simulink model "ImageProcessing"  (R2018b)
settings: Solver=FixedStepAuto  StartTime=0.0  StopTime=70  FixedStep=0.025  RelTol=1e-3  EnableMultiTasking=on
settings Model: Creator=barthal  LastModifiedBy=barthal
settings SolverCC: PositivePriorityOrder=on
settings DataIOCC: Decimation=5  SaveFormat=StructureWithTime
settings OptimizationCC: EnhancedBackFolding=on  PassReuseOutputArgsAs=Individual arguments  MaxStackSize=64  OptimizeBlockOrder=speed  DifferentSizesBufferReuse=on  OptimizationCustomize=off
settings DebuggingCC: ParameterTunabilityLossMsg=error
settings HardwareCC: ProdBitPerPointer=32  ProdBitPerSizeT=32  ProdBitPerPtrDiffT=32  ProdLargestAtomicInteger=Long  ProdLargestAtomicFloat=Double  ProdWordSize=32  ProdHWDeviceType=ARM Compatible->ARM Cortex
settings ModelReferenceCC: ModelReferenceNumInstancesAllowed=Single
settings RTWCC: SystemTargetFile=ert.tlc  HardwareBoard=Raspberry Pi  TLCOptions="-aInlineSetEventsForThisBaseRateFcn=TLC_FALSE -aSuppressMultiTaskScheduler=TLC_FALSE  -aRateBasedStepFcn=0"  GenCodeOnly=on  TemplateMakefile=ert_default_tmf  GenerateReport=on  Toolchain=GNU GCC Raspberry Pi  BuildConfiguration=Faster Runs  IncludeHyperlinkInReport=on  LaunchReport=on  TargetLang=C++  GenerateTraceInfo=on  GenerateTraceReport=on  GenerateTraceReportSl=on  GenerateTraceReportSf=on  GenerateTraceReportEml=on
settings CodeAppCC: ForceParamTrailComments=on  IgnoreCustomStorageClasses=off  OperatorAnnotations=on  SimulinkDataObjDesc=on  SFDataObjDesc=on  InsertBlockDesc=on
settings ERTTargetCC: TargetLangStandard=C++03 (ISO)  MatFileLogging=on  MultiInstanceERTCode=on  CodeInterfacePackaging=C++ class  SupportVariableSizeSignals=on  MultiInstanceErrorCode=Warning  RootIOFormat=Structure reference

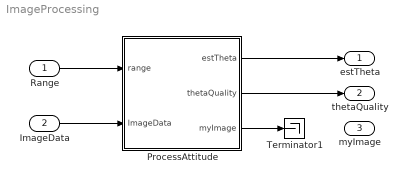
== system ImageProcessing ==
  Range : Inport  OutDataTypeStr=double  PortDimensions=4
  ImageData : Inport  Port=2  OutDataTypeStr=uint8  PortDimensions=[307200]
  ProcessAttitude : Subsystem
  Terminator1 : Terminator
  estTheta : Outport  OutDataTypeStr=double  PortDimensions=1
  thetaQuality : Outport  Port=2  OutDataTypeStr=double  PortDimensions=1
  myImage : Outport  Port=3  OutDataTypeStr=uint8
  wires:
  Range/1 -> ProcessAttitude/1(range)
  ImageData/1 -> ProcessAttitude/2(ImageData)
  ProcessAttitude/3(myImage) -> Terminator1/1
  ProcessAttitude/2(thetaQuality) -> thetaQuality/1
  ProcessAttitude/1(estTheta) -> estTheta/1

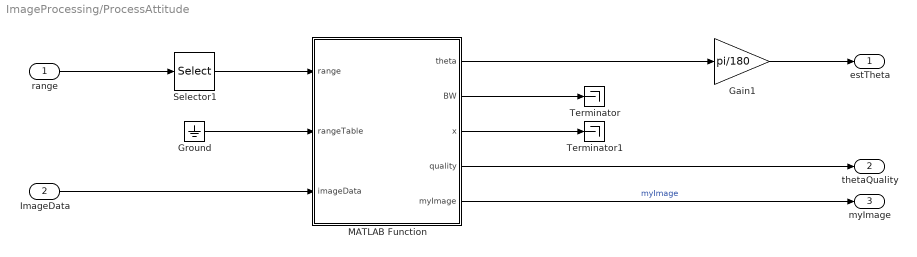
== system ImageProcessing/ProcessAttitude ==
  range : Inport  PortDimensions=4
  ImageData : Inport  Port=2  OutDataTypeStr=uint8  PortDimensions=[307200]
  Gain1 : Gain  Gain=pi/180
  Ground : Ground
  MATLAB Function : MATLAB Function  TreatAsAtomicUnit=on
  Selector1 : Selector  InputPortWidth=4  IndexOptions=Index vector (dialog)  Indices=1  OutputSizes=1
  Terminator : Terminator
  Terminator1 : Terminator
  estTheta : Outport
  thetaQuality : Outport  Port=2
  myImage : Outport  Port=3  OutDataTypeStr=uint8
  wires:
  MATLAB Function/3(x) -> Terminator1/1
  MATLAB Function/2(BW) -> Terminator/1
  MATLAB Function/5(myImage) -> myImage/1  "myImage"
  MATLAB Function/4(quality) -> thetaQuality/1
  MATLAB Function/1(theta) -> Gain1/1
  range/1 -> Selector1/1
  Selector1/1 -> MATLAB Function/1(range)
  Gain1/1 -> estTheta/1
  ImageData/1 -> MATLAB Function/3(imageData)
  Ground/1 -> MATLAB Function/2(rangeTable)

== matlab function ImageProcessing/ProcessAttitude/MATLAB Function ==
  data: range input; theta output; BW output; x output; quality output; rangeTable input; imageData input; myImage output uint8
function [theta,BW,x,quality,myImage] = callimageProcess(range,rangeTable,imageData)

% persistent camObj
% 
% if isempty(camObj)
%     adaptorname = 'winvideo';
%     camObj = imaq.VideoDevice(adaptorname);
% end

% Use this if importing a 3-channel color image
% b=imageData(:,1);
% g=imageData(:,2);
% r=imageData(:,3);
% 
% b2=reshape(b,640,480);
% g2=reshape(g,640,480);
% r2=reshape(r,640,480);
% 
% myImage = uint8(zeros(480,640,3));
% 
% myImage(:,:,1) = r2';
% myImage(:,:,2) = g2';
% myImage(:,:,3) = b2';

% Use this if importing a 1 channel grayscale image
inputImage=reshape(imageData,640,480);
% myImage = uint8(zeros(480,640));
myImage = inputImage';

% theta = 0;
% BW = 0;
% x = 0;
% quality = 0;
[theta,BW,x,quality] = imageProcess(myImage,range,rangeTable);
